simulink model "FunzioneDinamicaInversaSimulink"  (R2020b)
settings: Solver=VariableStepAuto  StartTime=0.0  StopTime=1  RelTol=1e-3
values from neighbouring files (symbols this model uses):
  theta1ldm = theta1 + Ldm_theta1.moto.data{1,1}.v    [PKM_main.m]
  theta1ldm_p = theta1_p + Ldm_theta1.moto.data{2,1}.v    [PKM_main.m]
  theta2ldm = theta2 + Ldm_theta2.moto.data{1,1}.v    [PKM_main.m]
  theta2ldm_p = theta2_p + Ldm_theta2.moto.data{2,1}.v    [PKM_main.m]
libraries: pid_lib x1
settings Model: Creator=daniele_ravasio  LastModifiedBy=daniele_ravasio

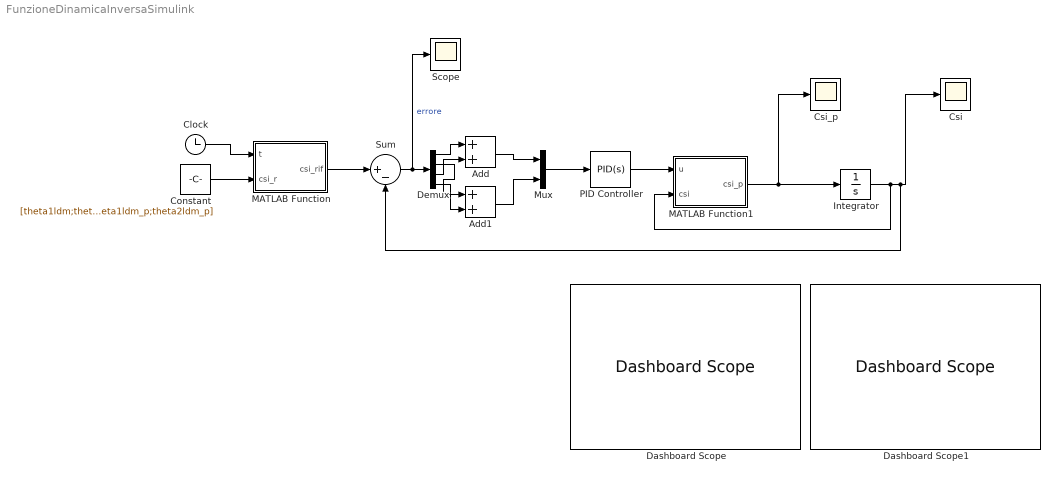
== system FunzioneDinamicaInversaSimulink ==
  Add : Sum
  Add1 : Sum
  Clock : Clock
  Constant : Constant  Value=[theta1ldm;theta2ldm;theta1ldm_p;theta2ldm_p]  VectorParams1D=off
  Csi : Scope
  Csi_p : Scope
  Dashboard Scope : DashboardScope
  Dashboard Scope1 : DashboardScope
  Demux : Demux
  Integrator : Integrator  InitialCondition=[theta1ldm(1,1),theta2ldm(1,1),theta1ldm_p(1,1),theta2ldm_p(1,1)]'
  MATLAB Function : MATLAB Function  TreatAsAtomicUnit=on
  MATLAB Function1 : MATLAB Function  TreatAsAtomicUnit=on
  Mux : Mux  Inputs=2
  PID Controller : pid_lib/PID Controller  Controller=PID  Form=Parallel  TimeDomain=Continuous-time  UseExternalTs=off  SampleTime=-1  IntegratorMethod=Forward Euler  FilterMethod=Forward Euler  ControllerParametersSource=internal  P=1  I=1  D=1  UseFilter=on  N=100  TunerSelectOption=Transfer Function Based (PID Tuner App)  InitialConditionSource=internal  InitialConditionForIntegrator=0  InitialConditionForFilter=0  DifferentiatorICPrevScaledInput=0  ExternalReset=none  TrackingMode=off  Kt=1  LimitOutput=off  SatLimitsSource=internal  UpperSaturationLimit=inf  LowerSaturationLimit=-inf  LinearizeAsGain=on  AntiWindupMode=none  Kb=1  POutMin=[]  POutMax=[]  IOutMin=[]  IOutMax=[]  DOutMin=[]  DOutMax=[]  NOutMin=[]  NOutMax=[]  SumOutMin=[]  SumOutMax=[]  SaturationOutMin=[]  SaturationOutMax=[]  PParamMin=[]  PParamMax=[]  IParamMin=[]  IParamMax=[]  DParamMin=[]  DParamMax=[]  NParamMin=[]  NParamMax=[]  KbParamMin=[]  KbParamMax=[]  KtParamMin=[]  KtParamMax=[]  KbOutMin=[]  KbOutMax=[]  KtOutMin=[]  KtOutMax=[]  IntegratorOutMin=[]  IntegratorOutMax=[]  FilterOutMin=[]  FilterOutMax=[]  SumI1OutMin=[]  SumI1OutMax=[]  SumI2OutMin=[]  SumI2OutMax=[]  SumI3OutMin=[]  SumI3OutMax=[]  SumI4OutMin=[]  SumI4OutMax=[]  SumDOutMin=[]  SumDOutMax=[]  DifferentiatorOutMin=[]  DifferentiatorOutMax=[]  FilterDiffOutCoefMin=[]  FilterDiffOutCoefMax=[]  ReciprocalOutMin=[]  ReciprocalOutMax=[]  SumDenOutMin=[]  SumDenOutMax=[]  SumNumOutMin=[]  SumNumOutMax=[]  DivideOutMin=[]  DivideOutMax=[]  UdiffTsProdOutMin=[]  UdiffTsProdOutMax=[]  NTsProdOutMin=[]  NTsProdOutMax=[]  UintegralTsProdOutMin=[]  UintegralTsProdOutMax=[]  UngainTsProdOutMin=[]  UngainTsProdOutMax=[]  IntegratorContinuousStateAttributes=''  IntegratorStateMustResolveToSignalObject=off  IntegratorRTWStateStorageClass=Auto  FilterContinuousStateAttributes=''  FilterStateMustResolveToSignalObject=off  FilterRTWStateStorageClass=Auto  ParallelPVariant=InternalParameters  IdealPVariant=Disabled  IVariant=InternalParameters  DVariant=InternalParameters  IntegratorVariant=Continuous  SatVariant=Disabled  AWVariant=Passthrough  PCopyVariant=Disabled  TRVariant=Disabled  FdbkBlocksVariant=Forward  IdealPFdbkVariant=Disabled  SatFdbkVariant=Disabled  DerivativeFilterVariant=ContFilter  NVariant=InternalParameters  NCopyVariant=Disabled  FilterICVariant=InternalICsFilter  IntegratorICVariant=InternalICs  ExternalResetVariant=Disabled  TRSumVariant=Passthrough  SumFdbkVariant=Disabled  SumVariant=Sum_PID  TsampFilterVariant=InternalTs  TsampNgainVariant=Passthrough  TsampIntegralVariant=Passthrough  ExternalSaturationOutDataTypeStr=Inherit: Same as second input
  Scope : Scope
  Sum : Sum  Inputs=|+-
  wires:
  Integrator/1 -> MATLAB Function1/2(csi), Csi/1, Sum/2
  MATLAB Function1/1(csi_p) -> Integrator/1, Csi_p/1
  PID Controller/1 -> MATLAB Function1/1(u)
  Sum/1 -> Scope/1, Demux/1  "errore"
  Demux/1 -> Add/1
  Demux/4 -> Add1/2
  Add/1 -> Mux/1
  Add1/1 -> Mux/2
  Mux/1 -> PID Controller/1
  Demux/3 -> Add/2
  Demux/2 -> Add1/1
  Clock/1 -> MATLAB Function/1(t)
  Constant/1 -> MATLAB Function/2(csi_r)
  MATLAB Function/1(csi_rif) -> Sum/1

== matlab function FunzioneDinamicaInversaSimulink/MATLAB Function ==
  data: t input; csi_rif output; csi_r input
function csi_rif = fcn(t,csi_r)


% tempo T, f(T), tempo di interpolazione (t) 
T = linspace(0,1,1000);
csi_rif = [interp1(T,csi_r(1,:),t);interp1(T,csi_r(2,:),t);interp1(T,csi_r(3,:),t);interp1(T,csi_r(4,:),t)];
%y_cap(2,:) = interp1(T,Tau(2,:),t);

== matlab function FunzioneDinamicaInversaSimulink/MATLAB Function1 ==
  data: u input; csi_p output; csi input
function csi_p = f(u,csi)

csi_p = F(u,csi);
